simulink model "test"  (R2024a)
settings: Solver=VariableStepAuto  StartTime=0.0  StopTime=inf  RelTol=1e-3
undefined symbols (not defined in the file): Angular, Linear
libraries: robotlib x2
settings Model: Creator=Fahim  LastModifiedBy=Fahim

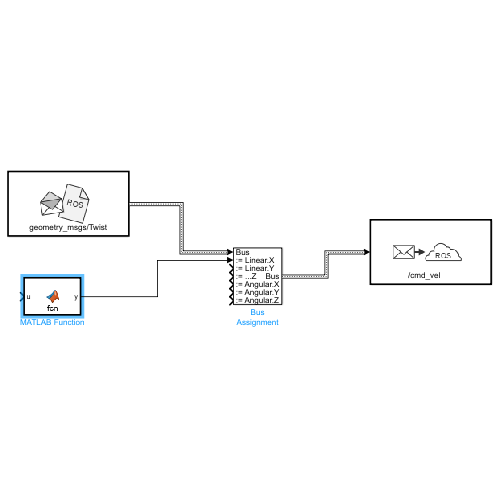
[thumbnail: Simulink's stored preview of the top-level diagram]
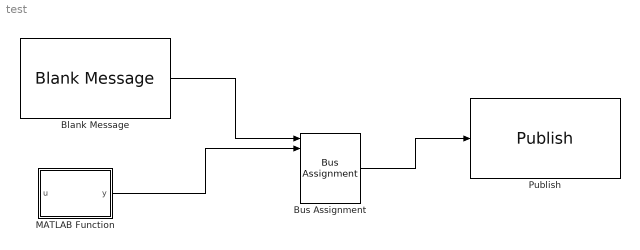
== system test ==
  Blank Message : robotlib/Blank Message  messageClass=Message  entityType=geometry_msgs/Twist  messageType=geometry_msgs/Twist  SampleTime=inf  legacyBusStruct=off
  Bus Assignment : BusAssignment  AssignedSignals=Linear.X,Linear.Y,Linear.Z,Angular.X,Angular.Y,Angular.Z
  MATLAB Function : MATLAB Function  TreatAsAtomicUnit=on
  Publish : robotlib/Publish  topicSource=Select from ROS network  topic=/cmd_vel  messageType=geometry_msgs/Twist  legacyBusStruct=off  messageQueueLength=1
  wires:
  Blank Message/1 -> Bus Assignment/1
  Bus Assignment/1 -> Publish/1
  MATLAB Function/1(y) -> Bus Assignment/2

== matlab function test/MATLAB Function ==
  data: u input; y output
function y = fcn(u)

y = 1;
